simulink model "GainDelay"  (R2024b)
settings: Solver=VariableStepAuto  StartTime=0.0  StopTime=10.0  RelTol=1e-3

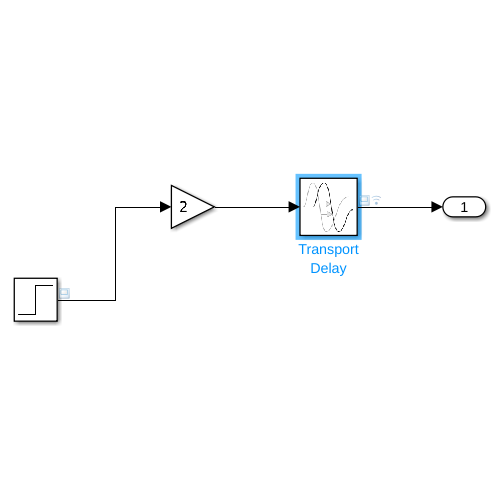
[thumbnail: Simulink's stored preview of the top-level diagram]
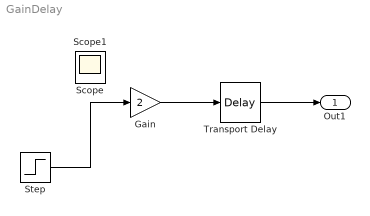
== system GainDelay ==
  Gain : Gain  Gain=2
  Step : Step  SampleTime=0
  Transport Delay : TransportDelay  DelayTime=4
  Out1 : Outport
  Scope : Scope
  Scope1 : Scope
  wires:
  Step/1 -> Gain/1
  Gain/1 -> Transport Delay/1
  Transport Delay/1 -> Out1/1
